simulink model "FullSystemSimFinal"  (R2020a)
settings: Solver=ode23t  StartTime=0.0  StopTime=T_sim  MaxStep=0.001  RelTol=1e-3
values from neighbouring files (symbols this model uses):
  a_friction = 0    [FullSystem.m]
  b_friction = 1.19    [FullSystem.m]
  C_T_matrix = ex2(2:12,2:12)'    [FullSystem.m]
  d_turbine = 0.15    [FullSystem.m]
  I_mp_data = ex4(:,5)    [FullSystem.m]
  I_sc_data = ex4(:,3)    [FullSystem.m]
  J_wind = 5.245e-6 * 1000    (= 0.005245)    [FullSystem.m]
  K_t = 0.023    [FullSystem.m]    (also in WindTurbine.m = 82.8991502528)
  K_v = 0.023 * pi / 30    (= 0.00240855436775)    [FullSystem.m]    (also in WindTurbine.m = 115.191730632)
  lambda_data_x = ex3(3, :)'    [FullSystem.m]
  lambda_opt = 2.8    [FullSystem.m]
  omega_0 = 1000    [FullSystem.m]    (also in SystemControl_script.m = 100:)
  P_max_EL = 3    [FullSystem.m]
  P_max_FC = 1    [FullSystem.m]
  R_LED_max = 75/4    (= 18.75)    [FullSystem.m]
  r_LED_x = ex1(4, :)'    [FullSystem.m]
  R_mp_data = ex4(:,6)    [FullSystem.m]
  r_PS_x = ex1(5,:)'    [FullSystem.m]
  r_solar_data_x = ex4(:,1)    [FullSystem.m]
  r_SP_x = ex1(3, :)'    [FullSystem.m]
  r_wind_data_x = ex3(1, :)'    [FullSystem.m]
  r_WT_x = ex1(2, :)'    [FullSystem.m]
  rho_air = 1.225    [FullSystem.m]
  step_size = T_sim/n    (= 0.01)    [FullSystem.m]
  t_sample = pwm_timer/10    (= 0.01)    [FullSystem.m]
  T_sim = 10    [FullSystem.m]    (also in SystemControl_script.m; model_1.m = 24)
  V_mp_data = ex4(:,4)    [FullSystem.m]
  V_oc_data = ex4(:,2)    [FullSystem.m]
  V_w_data_x = ex3(2,:)'    [FullSystem.m]
undefined symbols (not defined in the file or in its folder): DiscIntNeverNeededParam
libraries: fl_lib x68, nesl_utility x62, ee_lib x11, eePwmGenerator x4, simulink x2
(part 2 of 2)

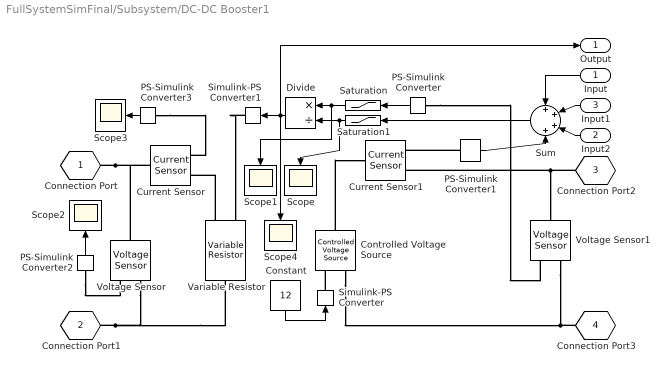
== system FullSystemSimFinal/Subsystem/DC-DC Booster1 ==
  Input : Inport
  Input2 : Inport  Port=2
  Input1 : Inport  Port=3
  Constant : Constant  Value=12
  Controlled Voltage Source : fl_lib/Electrical/Electrical Sources/Controlled Voltage Source
  Current Sensor : fl_lib/Electrical/Electrical Sensors/Current Sensor
  Current Sensor1 : fl_lib/Electrical/Electrical Sensors/Current Sensor
  Divide : Product  Inputs=*/
  PS-Simulink Converter{,1..3} (4 alike) : nesl_utility/PS-Simulink Converter  PhysicalDomain=network_engine_domain  SubClassName=ps_output  LeftPortType=input  RightPortType=output  PseudoPeriodic=off  Frequencies=[]  Unit=inherit  AffineConversion=off
  Saturation : Saturate  UpperLimit=13  LowerLimit=0
  Saturation1 : Saturate  UpperLimit=2  LowerLimit=0.01
  Scope{,1..4} (5 alike) : Scope
  Simulink-PS Converter : nesl_utility/Simulink-PS Converter  PhysicalDomain=network_engine_domain  SubClassName=ps_input  LeftPortType=input  RightPortType=output  PseudoPeriodic=off  Frequencies=[]  NoiseDistribution=none  NoiseParameters=[]  Unit=1  AffineConversion=off  FilteringAndDerivatives=provide  SimscapeFilterOrder=1  InputFilterTimeConstant=0.001  UdotUserProvided=0
  Simulink-PS Converter1 : nesl_utility/Simulink-PS Converter  PhysicalDomain=network_engine_domain  SubClassName=ps_input  LeftPortType=input  RightPortType=output  PseudoPeriodic=off  Frequencies=[]  NoiseDistribution=none  NoiseParameters=[]  Unit=1  AffineConversion=off  FilteringAndDerivatives=filter  SimscapeFilterOrder=1  InputFilterTimeConstant=0.001  UdotUserProvided=0
  Sum : Sum  Inputs=++++
  Variable Resistor : fl_lib/Electrical/Electrical Elements/Variable Resistor  Rmin=0 Ohm  i_specify=off  i_priority=None  i=0 A  i_nominal_specify=off  i_nominal_unit=A  i_nominal_value=1  v_specify=off  v_priority=None  v=0 V  v_nominal_specify=off  v_nominal_unit=V  v_nominal_value=1
  Voltage Sensor : fl_lib/Electrical/Electrical Sensors/Voltage Sensor
  Voltage Sensor1 : fl_lib/Electrical/Electrical Sensors/Voltage Sensor
  Connection Port : PMIOPort  Tag=PMCPort  Side=Left
  Connection Port1 : PMIOPort  Tag=PMCPort  Port=2  Side=Left
  Connection Port2 : PMIOPort  Tag=PMCPort  Port=3  Side=Right
  Connection Port3 : PMIOPort  Tag=PMCPort  Port=4  Side=Right
  Output : Outport
  wires:
  Constant/1 -> Simulink-PS Converter/1
  PS-Simulink Converter2/1 -> Scope2/1
  PS-Simulink Converter3/1 -> Scope3/1
  Saturation/1 -> Scope1/1, Divide/1
  PS-Simulink Converter/1 -> Saturation/1
  Saturation1/1 -> Scope/1, Divide/2
  Divide/1 -> Output/1, Scope4/1, Simulink-PS Converter1/1
  Sum/1 -> Saturation1/1
  PS-Simulink Converter1/1 -> Sum/4
  Input/1 -> Sum/1
  Input1/1 -> Sum/2
  Input2/1 -> Sum/3
  connections:
  Voltage Sensor1/RConn2 -- Controlled Voltage Source/RConn2 -- Connection Port3/RConn1
  Connection Port1/RConn1 -- Voltage Sensor/RConn2 -- Variable Resistor/RConn1
  Connection Port/RConn1 -- Current Sensor/LConn1 -- Voltage Sensor/LConn1
  Simulink-PS Converter1/RConn1 -- Variable Resistor/LConn1
  Simulink-PS Converter/RConn1 -- Controlled Voltage Source/RConn1
  PS-Simulink Converter1/LConn1 -- Current Sensor1/RConn1
  Variable Resistor/LConn2 -- Current Sensor/RConn2
  PS-Simulink Converter/LConn1 -- Voltage Sensor1/RConn1
  PS-Simulink Converter2/LConn1 -- Voltage Sensor/RConn1
  PS-Simulink Converter3/LConn1 -- Current Sensor/RConn1
  Controlled Voltage Source/LConn1 -- Current Sensor1/LConn1
  Connection Port2/RConn1 -- Current Sensor1/RConn2 -- Voltage Sensor1/LConn1

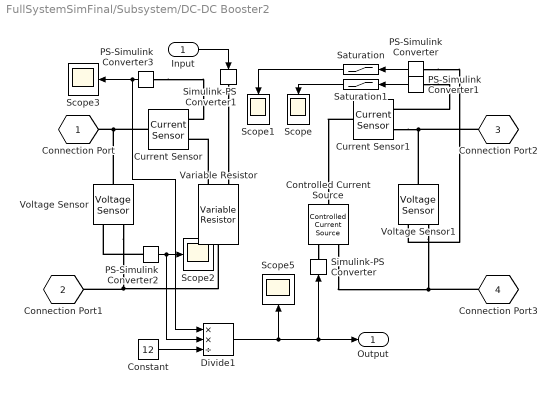
== system FullSystemSimFinal/Subsystem/DC-DC Booster2 ==
  Input : Inport
  Constant : Constant  Value=12
  Controlled Current Source : fl_lib/Electrical/Electrical Sources/Controlled Current Source
  Current Sensor : fl_lib/Electrical/Electrical Sensors/Current Sensor
  Current Sensor1 : fl_lib/Electrical/Electrical Sensors/Current Sensor
  Divide1 : Product  Inputs=**/
  PS-Simulink Converter{,1..3} (4 alike) : nesl_utility/PS-Simulink Converter  PhysicalDomain=network_engine_domain  SubClassName=ps_output  LeftPortType=input  RightPortType=output  PseudoPeriodic=off  Frequencies=[]  Unit=inherit  AffineConversion=off
  Saturation : Saturate  UpperLimit=13  LowerLimit=0
  Saturation1 : Saturate  UpperLimit=2  LowerLimit=0
  Scope{,1..3,5} (5 alike) : Scope
  Simulink-PS Converter : nesl_utility/Simulink-PS Converter  PhysicalDomain=network_engine_domain  SubClassName=ps_input  LeftPortType=input  RightPortType=output  PseudoPeriodic=off  Frequencies=[]  NoiseDistribution=none  NoiseParameters=[]  Unit=1  AffineConversion=off  FilteringAndDerivatives=filter  SimscapeFilterOrder=1  InputFilterTimeConstant=0.001  UdotUserProvided=0
  Simulink-PS Converter1 : nesl_utility/Simulink-PS Converter  PhysicalDomain=network_engine_domain  SubClassName=ps_input  LeftPortType=input  RightPortType=output  PseudoPeriodic=off  Frequencies=[]  NoiseDistribution=none  NoiseParameters=[]  Unit=1  AffineConversion=off  FilteringAndDerivatives=filter  SimscapeFilterOrder=1  InputFilterTimeConstant=0.001  UdotUserProvided=0
  Variable Resistor : fl_lib/Electrical/Electrical Elements/Variable Resistor  Rmin=0 Ohm  i_specify=off  i_priority=None  i=0 A  i_nominal_specify=off  i_nominal_unit=A  i_nominal_value=1  v_specify=off  v_priority=None  v=0 V  v_nominal_specify=off  v_nominal_unit=V  v_nominal_value=1
  Voltage Sensor : fl_lib/Electrical/Electrical Sensors/Voltage Sensor
  Voltage Sensor1 : fl_lib/Electrical/Electrical Sensors/Voltage Sensor
  Connection Port : PMIOPort  Tag=PMCPort  Side=Left
  Connection Port1 : PMIOPort  Tag=PMCPort  Port=2  Side=Left
  Connection Port2 : PMIOPort  Tag=PMCPort  Port=3  Side=Right
  Connection Port3 : PMIOPort  Tag=PMCPort  Port=4  Side=Right
  Output : Outport
  wires:
  Saturation/1 -> Scope1/1
  PS-Simulink Converter/1 -> Saturation/1
  PS-Simulink Converter1/1 -> Saturation1/1
  Saturation1/1 -> Scope/1
  Constant/1 -> Divide1/3
  PS-Simulink Converter2/1 -> Divide1/2, Scope2/1
  PS-Simulink Converter3/1 -> Scope3/1, Divide1/1
  Divide1/1 -> Output/1, Simulink-PS Converter/1, Scope5/1
  Input/1 -> Simulink-PS Converter1/1
  connections:
  Connection Port3/RConn1 -- Voltage Sensor1/RConn2 -- Controlled Current Source/RConn2
  Current Sensor1/RConn2 -- Connection Port2/RConn1 -- Voltage Sensor1/LConn1
  Voltage Sensor/RConn2 -- Variable Resistor/RConn1 -- Connection Port1/RConn1
  Current Sensor/LConn1 -- Voltage Sensor/LConn1 -- Connection Port/RConn1
  Simulink-PS Converter1/RConn1 -- Variable Resistor/LConn1
  Controlled Current Source/RConn1 -- Simulink-PS Converter/RConn1
  PS-Simulink Converter1/LConn1 -- Current Sensor1/RConn1
  Variable Resistor/LConn2 -- Current Sensor/RConn2
  PS-Simulink Converter/LConn1 -- Voltage Sensor1/RConn1
  PS-Simulink Converter2/LConn1 -- Voltage Sensor/RConn1
  PS-Simulink Converter3/LConn1 -- Current Sensor/RConn1
  Current Sensor1/LConn1 -- Controlled Current Source/LConn1

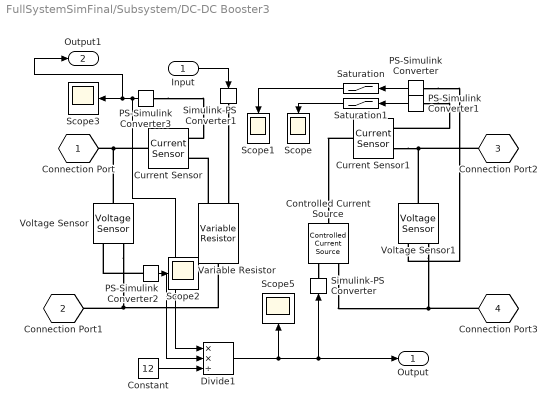
== system FullSystemSimFinal/Subsystem/DC-DC Booster3 ==
  Input : Inport
  Constant : Constant  Value=12
  Controlled Current Source : fl_lib/Electrical/Electrical Sources/Controlled Current Source
  Current Sensor : fl_lib/Electrical/Electrical Sensors/Current Sensor
  Current Sensor1 : fl_lib/Electrical/Electrical Sensors/Current Sensor
  Divide1 : Product  Inputs=**/
  PS-Simulink Converter{,1..3} (4 alike) : nesl_utility/PS-Simulink Converter  PhysicalDomain=network_engine_domain  SubClassName=ps_output  LeftPortType=input  RightPortType=output  PseudoPeriodic=off  Frequencies=[]  Unit=inherit  AffineConversion=off
  Saturation : Saturate  UpperLimit=13  LowerLimit=0
  Saturation1 : Saturate  UpperLimit=2  LowerLimit=0
  Scope{,1..3,5} (5 alike) : Scope
  Simulink-PS Converter : nesl_utility/Simulink-PS Converter  PhysicalDomain=network_engine_domain  SubClassName=ps_input  LeftPortType=input  RightPortType=output  PseudoPeriodic=off  Frequencies=[]  NoiseDistribution=none  NoiseParameters=[]  Unit=1  AffineConversion=off  FilteringAndDerivatives=filter  SimscapeFilterOrder=1  InputFilterTimeConstant=0.001  UdotUserProvided=0
  Simulink-PS Converter1 : nesl_utility/Simulink-PS Converter  PhysicalDomain=network_engine_domain  SubClassName=ps_input  LeftPortType=input  RightPortType=output  PseudoPeriodic=off  Frequencies=[]  NoiseDistribution=none  NoiseParameters=[]  Unit=1  AffineConversion=off  FilteringAndDerivatives=filter  SimscapeFilterOrder=1  InputFilterTimeConstant=0.001  UdotUserProvided=0
  Variable Resistor : fl_lib/Electrical/Electrical Elements/Variable Resistor  Rmin=0 Ohm  i_specify=off  i_priority=None  i=0 A  i_nominal_specify=off  i_nominal_unit=A  i_nominal_value=1  v_specify=off  v_priority=None  v=0 V  v_nominal_specify=off  v_nominal_unit=V  v_nominal_value=1
  Voltage Sensor : fl_lib/Electrical/Electrical Sensors/Voltage Sensor
  Voltage Sensor1 : fl_lib/Electrical/Electrical Sensors/Voltage Sensor
  Connection Port : PMIOPort  Tag=PMCPort  Side=Left
  Connection Port1 : PMIOPort  Tag=PMCPort  Port=2  Side=Left
  Connection Port2 : PMIOPort  Tag=PMCPort  Port=3  Side=Right
  Connection Port3 : PMIOPort  Tag=PMCPort  Port=4  Side=Right
  Output : Outport
  Output1 : Outport  Port=2
  wires:
  Saturation/1 -> Scope1/1
  PS-Simulink Converter/1 -> Saturation/1
  PS-Simulink Converter1/1 -> Saturation1/1
  Saturation1/1 -> Scope/1
  Constant/1 -> Divide1/3
  PS-Simulink Converter2/1 -> Divide1/2, Scope2/1
  PS-Simulink Converter3/1 -> Output1/1, Scope3/1, Divide1/1
  Input/1 -> Simulink-PS Converter1/1
  Divide1/1 -> Output/1, Simulink-PS Converter/1, Scope5/1
  connections:
  Connection Port3/RConn1 -- Voltage Sensor1/RConn2 -- Controlled Current Source/RConn2
  Current Sensor1/RConn2 -- Connection Port2/RConn1 -- Voltage Sensor1/LConn1
  Voltage Sensor/RConn2 -- Variable Resistor/RConn1 -- Connection Port1/RConn1
  Current Sensor/LConn1 -- Voltage Sensor/LConn1 -- Connection Port/RConn1
  Simulink-PS Converter1/RConn1 -- Variable Resistor/LConn1
  Controlled Current Source/RConn1 -- Simulink-PS Converter/RConn1
  PS-Simulink Converter1/LConn1 -- Current Sensor1/RConn1
  Variable Resistor/LConn2 -- Current Sensor/RConn2
  PS-Simulink Converter/LConn1 -- Voltage Sensor1/RConn1
  PS-Simulink Converter2/LConn1 -- Voltage Sensor/RConn1
  PS-Simulink Converter3/LConn1 -- Current Sensor/RConn1
  Current Sensor1/LConn1 -- Controlled Current Source/LConn1

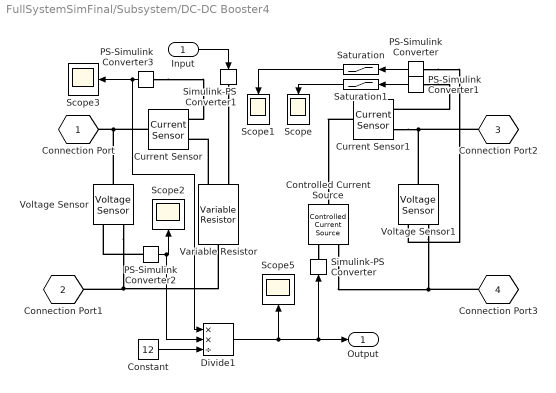
== system FullSystemSimFinal/Subsystem/DC-DC Booster4 ==
  Input : Inport
  Constant : Constant  Value=12
  Controlled Current Source : fl_lib/Electrical/Electrical Sources/Controlled Current Source
  Current Sensor : fl_lib/Electrical/Electrical Sensors/Current Sensor
  Current Sensor1 : fl_lib/Electrical/Electrical Sensors/Current Sensor
  Divide1 : Product  Inputs=**/
  PS-Simulink Converter{,1..3} (4 alike) : nesl_utility/PS-Simulink Converter  PhysicalDomain=network_engine_domain  SubClassName=ps_output  LeftPortType=input  RightPortType=output  PseudoPeriodic=off  Frequencies=[]  Unit=inherit  AffineConversion=off
  Saturation : Saturate  UpperLimit=13  LowerLimit=0
  Saturation1 : Saturate  UpperLimit=2  LowerLimit=0
  Scope{,1..3,5} (5 alike) : Scope
  Simulink-PS Converter : nesl_utility/Simulink-PS Converter  PhysicalDomain=network_engine_domain  SubClassName=ps_input  LeftPortType=input  RightPortType=output  PseudoPeriodic=off  Frequencies=[]  NoiseDistribution=none  NoiseParameters=[]  Unit=1  AffineConversion=off  FilteringAndDerivatives=filter  SimscapeFilterOrder=1  InputFilterTimeConstant=0.001  UdotUserProvided=0
  Simulink-PS Converter1 : nesl_utility/Simulink-PS Converter  PhysicalDomain=network_engine_domain  SubClassName=ps_input  LeftPortType=input  RightPortType=output  PseudoPeriodic=off  Frequencies=[]  NoiseDistribution=none  NoiseParameters=[]  Unit=1  AffineConversion=off  FilteringAndDerivatives=filter  SimscapeFilterOrder=1  InputFilterTimeConstant=0.001  UdotUserProvided=0
  Variable Resistor : fl_lib/Electrical/Electrical Elements/Variable Resistor  Rmin=0 Ohm  i_specify=off  i_priority=None  i=0 A  i_nominal_specify=off  i_nominal_unit=A  i_nominal_value=1  v_specify=off  v_priority=None  v=0 V  v_nominal_specify=off  v_nominal_unit=V  v_nominal_value=1
  Voltage Sensor : fl_lib/Electrical/Electrical Sensors/Voltage Sensor
  Voltage Sensor1 : fl_lib/Electrical/Electrical Sensors/Voltage Sensor
  Connection Port : PMIOPort  Tag=PMCPort  Side=Left
  Connection Port1 : PMIOPort  Tag=PMCPort  Port=2  Side=Left
  Connection Port2 : PMIOPort  Tag=PMCPort  Port=3  Side=Right
  Connection Port3 : PMIOPort  Tag=PMCPort  Port=4  Side=Right
  Output : Outport
  wires:
  Saturation/1 -> Scope1/1
  PS-Simulink Converter/1 -> Saturation/1
  PS-Simulink Converter1/1 -> Saturation1/1
  Saturation1/1 -> Scope/1
  Constant/1 -> Divide1/3
  PS-Simulink Converter2/1 -> Divide1/2, Scope2/1
  PS-Simulink Converter3/1 -> Scope3/1, Divide1/1
  Divide1/1 -> Simulink-PS Converter/1, Output/1, Scope5/1
  Input/1 -> Simulink-PS Converter1/1
  connections:
  Connection Port3/RConn1 -- Voltage Sensor1/RConn2 -- Controlled Current Source/RConn2
  Current Sensor1/RConn2 -- Connection Port2/RConn1 -- Voltage Sensor1/LConn1
  Voltage Sensor/RConn2 -- Variable Resistor/RConn1 -- Connection Port1/RConn1
  Current Sensor/LConn1 -- Voltage Sensor/LConn1 -- Connection Port/RConn1
  Simulink-PS Converter1/RConn1 -- Variable Resistor/LConn1
  Controlled Current Source/RConn1 -- Simulink-PS Converter/RConn1
  PS-Simulink Converter1/LConn1 -- Current Sensor1/RConn1
  Variable Resistor/LConn2 -- Current Sensor/RConn2
  PS-Simulink Converter/LConn1 -- Voltage Sensor1/RConn1
  PS-Simulink Converter2/LConn1 -- Voltage Sensor/RConn1
  PS-Simulink Converter3/LConn1 -- Current Sensor/RConn1
  Current Sensor1/LConn1 -- Controlled Current Source/LConn1

== system FullSystemSimFinal/Subsystem/Subsystem5 ==
  In1 : Inport
  Controlled PWM Voltage1 : ee_lib/Integrated Circuits/Controlled PWM Voltage  F=10 Hz  TD=0 s  pulse_width_offset=0 s  pulse_min=0 s  Vmin=0 V  Vmax=5 V  Vm=5 V  pwm_or_av=1  event_type=1  sample_time=1e-6 s  u_min=0  u_max=1
      settings: InternalSimscapePortConfiguration="{\"Bottom\":[],\"Left\":[{\"id\":\"u\",\"label\":\"u\",\"type\":\"input\"}],\"Right\":[{\"id\":\"p2\",\"label\":\"PWM\",\"type\":\"foundation.electrical.electrical\"},{\"id\":\"n2\",\"label\":\"REF\",\"type\":\"foundation.electrical.electrical\"}],\"Top\":[]}"
  Electrical Reference2 : fl_lib/Electrical/Electrical Elements/Electrical Reference
  PS-Simulink Converter4 : nesl_utility/PS-Simulink Converter  PhysicalDomain=network_engine_domain  SubClassName=ps_output  LeftPortType=input  RightPortType=output  PseudoPeriodic=off  Frequencies=[]  Unit=inherit  AffineConversion=off
  PWM Generator1 : eePwmGenerator/PWM Generator  CarrCount=Up  Tper=pwm_timer  Ts=t_sample
  Scope4 : Scope
  Simulink-PS Converter2 : nesl_utility/Simulink-PS Converter  PhysicalDomain=network_engine_domain  SubClassName=ps_input  LeftPortType=input  RightPortType=output  PseudoPeriodic=off  Frequencies=[]  NoiseDistribution=none  NoiseParameters=[]  Unit=1  AffineConversion=off  FilteringAndDerivatives=provide  SimscapeFilterOrder=1  InputFilterTimeConstant=0.001  UdotUserProvided=0
  Voltage Sensor2 : fl_lib/Electrical/Electrical Sensors/Voltage Sensor
  Conn1 : PMIOPort  Side=Right
  wires:
  In1/1 -> PWM Generator1/1
  PWM Generator1/1 -> Simulink-PS Converter2/1
  PS-Simulink Converter4/1 -> Scope4/1
  connections:
  PS-Simulink Converter4/LConn1 -- Voltage Sensor2/RConn1
  Voltage Sensor2/RConn2 -- Electrical Reference2/LConn1 -- Controlled PWM Voltage1/RConn2
  Voltage Sensor2/LConn1 -- Controlled PWM Voltage1/RConn1 -- Conn1/RConn1
  Simulink-PS Converter2/RConn1 -- Controlled PWM Voltage1/LConn1

== system FullSystemSimFinal/Subsystem/Subsystem6 ==
  In1 : Inport
  Controlled PWM Voltage1 : ee_lib/Integrated Circuits/Controlled PWM Voltage  F=10 Hz  TD=0 s  pulse_width_offset=0 s  pulse_min=0 s  Vmin=0 V  Vmax=5 V  Vm=5 V  pwm_or_av=1  event_type=1  sample_time=1e-6 s  u_min=0  u_max=1
      settings: InternalSimscapePortConfiguration="{\"Bottom\":[],\"Left\":[{\"id\":\"u\",\"label\":\"u\",\"type\":\"input\"}],\"Right\":[{\"id\":\"p2\",\"label\":\"PWM\",\"type\":\"foundation.electrical.electrical\"},{\"id\":\"n2\",\"label\":\"REF\",\"type\":\"foundation.electrical.electrical\"}],\"Top\":[]}"
  PS-Simulink Converter4 : nesl_utility/PS-Simulink Converter  PhysicalDomain=network_engine_domain  SubClassName=ps_output  LeftPortType=input  RightPortType=output  PseudoPeriodic=off  Frequencies=[]  Unit=inherit  AffineConversion=off
  PWM Generator1 : eePwmGenerator/PWM Generator  CarrCount=Up  Tper=pwm_timer  Ts=t_sample
  Scope4 : Scope
  Simulink-PS Converter2 : nesl_utility/Simulink-PS Converter  PhysicalDomain=network_engine_domain  SubClassName=ps_input  LeftPortType=input  RightPortType=output  PseudoPeriodic=off  Frequencies=[]  NoiseDistribution=none  NoiseParameters=[]  Unit=1  AffineConversion=off  FilteringAndDerivatives=provide  SimscapeFilterOrder=1  InputFilterTimeConstant=0.001  UdotUserProvided=0
  Voltage Sensor2 : fl_lib/Electrical/Electrical Sensors/Voltage Sensor
  Conn1 : PMIOPort  Side=Right
  Conn2 : PMIOPort  Port=2  Side=Right
  wires:
  In1/1 -> PWM Generator1/1
  PWM Generator1/1 -> Simulink-PS Converter2/1
  PS-Simulink Converter4/1 -> Scope4/1
  connections:
  PS-Simulink Converter4/LConn1 -- Voltage Sensor2/RConn1
  Voltage Sensor2/RConn2 -- Conn2/RConn1 -- Controlled PWM Voltage1/RConn2
  Voltage Sensor2/LConn1 -- Controlled PWM Voltage1/RConn1 -- Conn1/RConn1
  Simulink-PS Converter2/RConn1 -- Controlled PWM Voltage1/LConn1

== system FullSystemSimFinal/Subsystem/Subsystem7 ==
  In1 : Inport
  Controlled PWM Voltage2 : ee_lib/Integrated Circuits/Controlled PWM Voltage  F=10 Hz  TD=0 s  pulse_width_offset=0 s  pulse_min=0 s  Vmin=0 V  Vmax=5 V  Vm=5 V  pwm_or_av=1  event_type=1  sample_time=1e-6 s  u_min=0  u_max=1
      settings: InternalSimscapePortConfiguration="{\"Bottom\":[],\"Left\":[{\"id\":\"u\",\"label\":\"u\",\"type\":\"input\"}],\"Right\":[{\"id\":\"p2\",\"label\":\"PWM\",\"type\":\"foundation.electrical.electrical\"},{\"id\":\"n2\",\"label\":\"REF\",\"type\":\"foundation.electrical.electrical\"}],\"Top\":[]}"
  PS-Simulink Converter6 : nesl_utility/PS-Simulink Converter  PhysicalDomain=network_engine_domain  SubClassName=ps_output  LeftPortType=input  RightPortType=output  PseudoPeriodic=off  Frequencies=[]  Unit=inherit  AffineConversion=off
  PWM Generator2 : eePwmGenerator/PWM Generator  CarrCount=Up  Tper=pwm_timer  Ts=t_sample
  Scope6 : Scope
  Simulink-PS Converter3 : nesl_utility/Simulink-PS Converter  PhysicalDomain=network_engine_domain  SubClassName=ps_input  LeftPortType=input  RightPortType=output  PseudoPeriodic=off  Frequencies=[]  NoiseDistribution=none  NoiseParameters=[]  Unit=1  AffineConversion=off  FilteringAndDerivatives=provide  SimscapeFilterOrder=1  InputFilterTimeConstant=0.001  UdotUserProvided=0
  Voltage Sensor4 : fl_lib/Electrical/Electrical Sensors/Voltage Sensor
  Conn1 : PMIOPort  Side=Right
  Conn2 : PMIOPort  Port=2  Side=Right
  wires:
  PWM Generator2/1 -> Simulink-PS Converter3/1
  In1/1 -> PWM Generator2/1
  PS-Simulink Converter6/1 -> Scope6/1
  connections:
  Voltage Sensor4/LConn1 -- Controlled PWM Voltage2/RConn1 -- Conn1/RConn1
  Voltage Sensor4/RConn2 -- Conn2/RConn1 -- Controlled PWM Voltage2/RConn2
  PS-Simulink Converter6/LConn1 -- Voltage Sensor4/RConn1
  Simulink-PS Converter3/RConn1 -- Controlled PWM Voltage2/LConn1

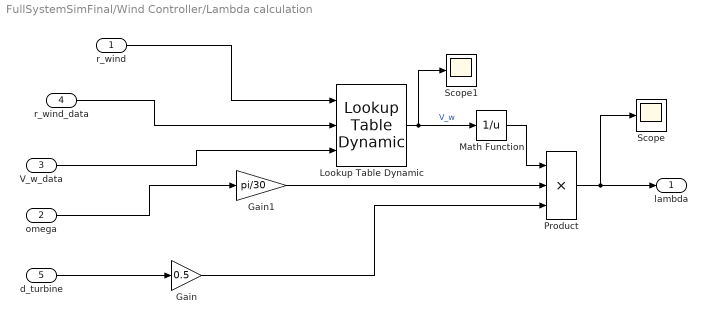
== system FullSystemSimFinal/Wind Controller/Lambda calculation ==
  r_wind : Inport
  omega : Inport  Port=2
  V_w_data : Inport  Port=3
  r_wind_data : Inport  Port=4
  d_turbine : Inport  Port=5
  Gain : Gain  Gain=0.5
  Gain1 : Gain  Gain=pi/30
  Lookup Table Dynamic : simulink/Lookup Tables/Lookup Table Dynamic  LookUpMeth=Interpolation-Use End Values  OutDataType=fixdt('double')  OutScaling=[]  OutputDataTypeScalingMode=Specify via dialog  OutDataTypeStr=double  DoSatur=off
  Math Function : Math  Operator=reciprocal  SignedPower=on  SaturateOnIntegerOverflow=on
  Product : Product  Inputs=3
  Scope : Scope
  Scope1 : Scope
  lambda : Outport
  wires:
  r_wind_data/1 -> Lookup Table Dynamic/2
  Product/1 -> Scope/1, lambda/1
  d_turbine/1 -> Gain/1
  V_w_data/1 -> Lookup Table Dynamic/3
  Math Function/1 -> Product/1
  r_wind/1 -> Lookup Table Dynamic/1
  omega/1 -> Gain1/1
  Lookup Table Dynamic/1 -> Scope1/1, Math Function/1  "V_w"
  Gain/1 -> Product/3
  Gain1/1 -> Product/2

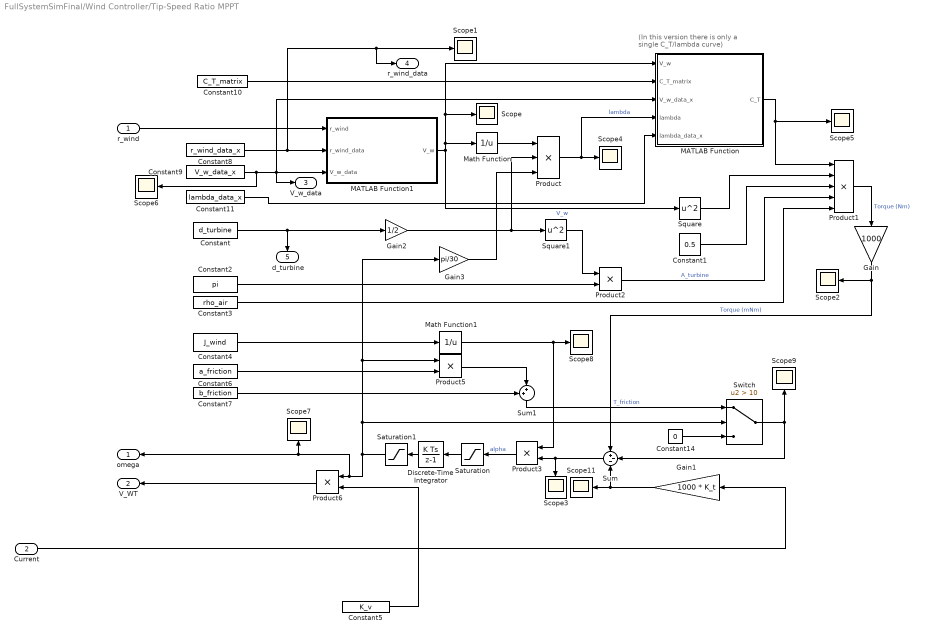
== system FullSystemSimFinal/Wind Controller/Tip-Speed Ratio MPPT ==
  note: (In this version there is only
      | a single C_T/lambda curve)
  r_wind : Inport
  Current : Inport  Port=2
  Constant : Constant  Value=d_turbine
  Constant1 : Constant  Value=0.5
  Constant10 : Constant  Value=C_T_matrix
  Constant11 : Constant  Value=lambda_data_x
  Constant14 : Constant  Value=0
  Constant2 : Constant  Value=pi
  Constant3 : Constant  Value=rho_air
  Constant4 : Constant  Value=J_wind  SampleTime=step_size
  Constant5 : Constant  Value=K_v
  Constant6 : Constant  Value=a_friction
  Constant7 : Constant  Value=b_friction  SampleTime=step_size
  Constant8 : Constant  Value=r_wind_data_x
  Constant9 : Constant  Value=V_w_data_x
  Discrete-Time Integrator : DiscreteIntegrator  InitialCondition=omega_0  SampleTime=-1  ICPrevOutput=DiscIntNeverNeededParam  ICPrevScaledInput=DiscIntNeverNeededParam
  Gain : Gain  Gain=1000
  Gain1 : Gain  Gain=1000 * K_t
  Gain2 : Gain  Gain=1/2
  Gain3 : Gain  Gain=pi/30
  MATLAB Function : MATLAB Function  TreatAsAtomicUnit=on
  MATLAB Function1 : MATLAB Function  TreatAsAtomicUnit=on
  Math Function : Math  Operator=reciprocal  SignedPower=on  SaturateOnIntegerOverflow=on
  Math Function1 : Math  Operator=reciprocal  SignedPower=on  SaturateOnIntegerOverflow=on
  Product : Product  Inputs=3
  Product1 : Product  Inputs=5
  Product{2..3,5..6} (4 alike) : Product
  Saturation : Saturate  UpperLimit=10000  LowerLimit=-10000
  Saturation1 : Saturate  UpperLimit=3000  LowerLimit=1000
  Scope{,1..9,11} (11 alike) : Scope
  Square : Math  Operator=square  SignedPower=on  SaturateOnIntegerOverflow=on
  Square1 : Math  Operator=square  SignedPower=on  SaturateOnIntegerOverflow=on
  Sum : Sum  Inputs=+--
  Sum1 : Sum  Inputs=++|
  Switch : Switch  Criteria=u2 > Threshold  Threshold=10
  omega : Outport
  V_WT : Outport  Port=2
  V_w_data : Outport  Port=3
  r_wind_data : Outport  Port=4
  d_turbine : Outport  Port=5
  wires:
  Switch/1 -> Scope9/1, Sum/2
  Gain1/1 -> Sum/3, Scope11/1
  Product3/1 -> Saturation/1  "alpha"
  Math Function/1 -> Product/1
  Constant10/1 -> MATLAB Function/2(C_T_matrix)
  Product2/1 -> Product1/4  "A_turbine"
  Constant5/1 -> Product6/2
  Math Function1/1 -> Product3/1, Scope8/1
  Constant6/1 -> Product5/2
  Sum/1 -> Product3/2, Scope3/1
  Constant2/1 -> Product2/2
  Current/1 -> Gain1/1
  Constant4/1 -> Math Function1/1
  Square/1 -> Product1/2
  Constant3/1 -> Product1/5
  Constant7/1 -> Sum1/1
  r_wind/1 -> MATLAB Function1/1(r_wind)
  Product/1 -> MATLAB Function/4(lambda), Scope4/1  "lambda"
  Constant/1 -> Gain2/1, d_turbine/1
  Constant8/1 -> r_wind_data/1, Scope1/1, MATLAB Function1/2(r_wind_data)
  Constant9/1 -> Scope6/1, V_w_data/1, MATLAB Function/3(V_w_data_x), MATLAB Function1/3(V_w_data)
  Product6/1 -> V_WT/1
  Square1/1 -> Product2/1
  MATLAB Function/1(C_T) -> Product1/1, Scope5/1
  Gain/1 -> Scope2/1, Sum/1  "Torque (mNm)"
  Product5/1 -> Sum1/2
  Constant11/1 -> MATLAB Function/5(lambda_data_x)
  Constant14/1 -> Switch/3
  Saturation/1 -> Discrete-Time Integrator/1
  Constant1/1 -> Product1/3
  Sum1/1 -> Switch/1  "T_friction"
  Product1/1 -> Gain/1  "Torque (Nm)"
  MATLAB Function1/1(V_w) -> MATLAB Function/1(V_w), Scope/1, Math Function/1, Square/1  "V_w"
  Gain2/1 -> Square1/1, Product/2
  Gain3/1 -> Product/3
  Saturation1/1 -> Switch/2, Gain3/1, Product5/1, Scope7/1, omega/1, Product6/1
  Discrete-Time Integrator/1 -> Saturation1/1

== matlab function FullSystemSimFinal/Wind Controller/Tip-Speed Ratio MPPT/MATLAB Function1 ==
  data: r_wind input; V_w output; r_wind_data input; V_w_data input
function V_w = TableLookup(r_wind,r_wind_data,V_w_data)

V_w = interp1(r_wind_data,V_w_data,min(r_wind,0.999999));

== matlab function FullSystemSimFinal/Wind Controller/Tip-Speed Ratio MPPT/MATLAB Function ==
  data: V_w input; C_T output; C_T_matrix input; V_w_data_x input; lambda input; lambda_data_x input
function C_T = MatrixLookUp(V_w,C_T_matrix,V_w_data_x,lambda,lambda_data_x)

lambda = min( max(lambda, 0), 10);

C_T = interp1(lambda_data_x,interp1(V_w_data_x,C_T_matrix,V_w),lambda);

== matlab function FullSystemSimFinal/Subsystem1/MATLAB Function ==
  data: r_SP input; I_SP output; R_load input; r_solar_data input; V_oc_data input; I_sc_data input; V_mp_data input; I_mp_data input; R_mp_data input
function I_SP = SolarInterp(r_SP,R_load, r_solar_data, V_oc_data, I_sc_data, V_mp_data, I_mp_data, R_mp_data)
V_oc = interp1(r_solar_data,V_oc_data,r_SP);
I_sc = interp1(r_solar_data,I_sc_data,r_SP);
V_mp = interp1(r_solar_data,V_mp_data,r_SP);
I_mp = interp1(r_solar_data,I_mp_data,r_SP);
R_mp = interp1(r_solar_data,R_mp_data,r_SP);

if (R_load < R_mp )
    I_SP = max(I_sc/((1/R_load)+((I_sc-I_mp)/V_mp)) / R_load, 0);
else
    I_SP = max((I_mp+I_mp*V_mp/(V_oc-V_mp))/((1/R_load)+I_mp/(V_oc-V_mp)) / R_load, 0);
end
